simulink model "hil"  (R2025b)
settings: Solver=ode2  StartTime=0.0  StopTime=100  FixedStep=0.0025  RelTol=1e-3
undefined symbols (not defined in the file or in its folder): LF
libraries: instrumentseriallib x3
settings Model: SimulationMode=accelerator  PauseTimes=16  Creator=joedo  LastModifiedBy=trist
settings SFSimCC: SimHardwareAcceleration=native

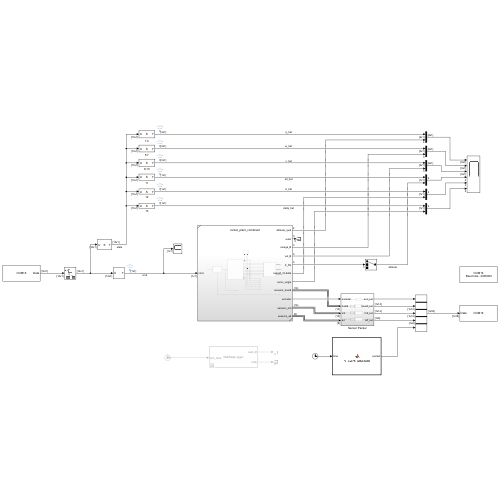
[thumbnail: Simulink's stored preview of the top-level diagram]
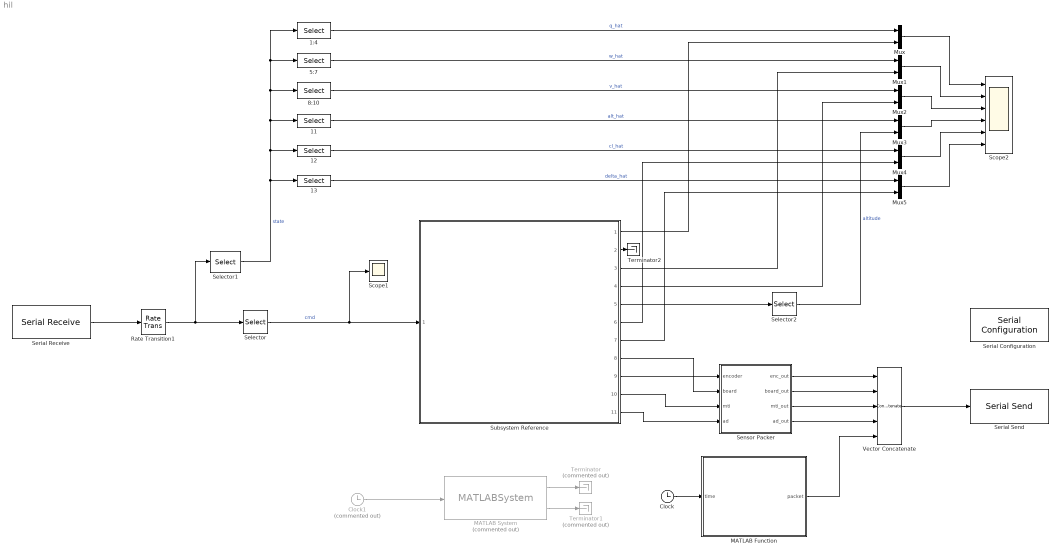
== system hil ==
  11 : Selector  InputPortWidth=13  IndexOptions=Index vector (dialog)  Indices=[11]  OutputSizes=1
  12 : Selector  InputPortWidth=13  IndexOptions=Index vector (dialog)  Indices=[12]  OutputSizes=1
  13 : Selector  InputPortWidth=13  IndexOptions=Index vector (dialog)  Indices=[13]  OutputSizes=1
  1:4 : Selector  InputPortWidth=13  IndexOptions=Index vector (dialog)  Indices=[1:4]  OutputSizes=1
  5:7 : Selector  InputPortWidth=13  IndexOptions=Index vector (dialog)  Indices=[5:7]  OutputSizes=1
  8:10 : Selector  InputPortWidth=13  IndexOptions=Index vector (dialog)  Indices=[8:10]  OutputSizes=1
  Clock : Clock
  Clock1 : Clock  Commented=on
  MATLAB Function : MATLAB Function  TreatAsAtomicUnit=on
  MATLAB System : MATLABSystem  Commented=on  System=WallStepLogger  Ts=0.0025  MaxSamples=50000  FileName=wall_step_log.mat  SimulateUsing=Code generation
      mask Type: WallStepLogger
  Mux{,1..5} (6 alike) : Mux  Inputs=2
  Rate Transition1 : RateTransition  OutPortSampleTime=0.01
  Scope1 : Scope
      settings: ActiveDisplayYMinimum=-1  ActiveDisplayYMaximum=1  DataLoggingVariableName=proccmd
  Scope2 : Scope  NumInputPorts=6
      settings: ActiveDisplayString=6  ActiveDisplayYMinimum=-0.00021816615649929114  ActiveDisplayYMaximum=0.0019634954084936209  DataLoggingVariableName=ScopeData9
  Selector : Selector  InputPortWidth=14  IndexOptions=Index vector (dialog)  Indices=[1]  OutputSizes=1
  Selector1 : Selector  InputPortWidth=14  IndexOptions=Index vector (dialog)  Indices=[2:14]  OutputSizes=1
  Selector2 : Selector  InputPortWidth=3  IndexOptions=Index vector (dialog)  Indices=[1]  OutputSizes=1
  Sensor Packer : Subsystem
  Serial Configuration : instrumentseriallib/Serial Configuration  Priority=-200000  PortSel=COM16  Port=COM16  ComPort=COM16  BaudRate=2000000  DataBits=8  Parity=none  StopBits=1  ByteOrder=little-endian  FlowControl=none  Timeout=10  SimulateUsing=Interpreted execution  BlockInModel=on  aMode=1
  Serial Receive : instrumentseriallib/Serial Receive  Priority=1  PortSel=COM16  Port=COM16  ComPort=COM16  DataType=double  SaveDataType=uint8  ToggleHeader=on  Header=[111, 114, 122, 33]  ToggleDataSize=on  DataSize=[14]  ToggleTerminator=on  Terminator=LF ('\n')  CustomTerminator=[]  InputFormat=Column major  EnableBlockingMode=on  ActionDataUnavailable=Output last received value  ActionWhenDataUnavailable=Output last received value  CustomValue=0  SampleTime=0.0025  SimulateUsing=Interpreted execution  BlockInModel=on  aMode=1  LibraryInUse=instrumentlib
  Serial Send : instrumentseriallib/Serial Send  Priority=1  PortSel=COM16  Port=COM16  ComPort=COM16  Header=[111, 114, 122, 33]  Terminator=LF ('\n')  CustomTerminator=[]  EnableBlockingMode=off  SimulateUsing=Interpreted execution  BlockInModel=on  aMode=1
  Subsystem Reference : Subsystem  ReferencedSubsystem=rocket_plant_combined
  Terminator : Terminator  Commented=on
  Terminator1 : Terminator  Commented=on
  Terminator2 : Terminator
  Vector Concatenate : Concatenate  NumInputs=5
  wires:
  Vector Concatenate/1 -> Serial Send/1
  Selector/1 -> Scope1/1, Subsystem Reference/1  "cmd"
  Selector1/1 -> 13/1, 12/1, 11/1, 8:10/1, 5:7/1, 1:4/1  "state"
  1:4/1 -> Mux/1  "q_hat"
  5:7/1 -> Mux1/1  "w_hat"
  8:10/1 -> Mux2/1  "v_hat"
  11/1 -> Mux3/1  "alt_hat"
  12/1 -> Mux4/1  "cl_hat"
  13/1 -> Mux5/1  "delta_hat"
  Subsystem Reference/1 -> Mux/2
  Subsystem Reference/3 -> Mux1/2
  Subsystem Reference/4 -> Mux2/2
  Subsystem Reference/5 -> Selector2/1
  Selector2/1 -> Mux3/2  "altitude"
  Subsystem Reference/6 -> Mux4/2
  Subsystem Reference/7 -> Mux5/2
  Mux/1 -> Scope2/1
  Mux1/1 -> Scope2/2
  Mux2/1 -> Scope2/3
  Mux3/1 -> Scope2/4
  Mux4/1 -> Scope2/5
  Mux5/1 -> Scope2/6
  Rate Transition1/1 -> Selector1/1, Selector/1
  Clock/1 -> MATLAB Function/1(time)
  MATLAB Function/1(packet) -> Vector Concatenate/5
  Serial Receive/1 -> Rate Transition1/1
  Clock1/1 -> MATLAB System/1
  MATLAB System/1 -> Terminator/1
  MATLAB System/2 -> Terminator1/1
  Subsystem Reference/2 -> Terminator2/1
  Sensor Packer/2(board_out) -> Vector Concatenate/2
  Sensor Packer/1(enc_out) -> Vector Concatenate/1
  Sensor Packer/3(mti_out) -> Vector Concatenate/3
  Sensor Packer/4(ad_out) -> Vector Concatenate/4
  Subsystem Reference/9 -> Sensor Packer/1(encoder)
  Subsystem Reference/8 -> Sensor Packer/2(board)
  Subsystem Reference/10 -> Sensor Packer/3(mti)
  Subsystem Reference/11 -> Sensor Packer/4(ad)

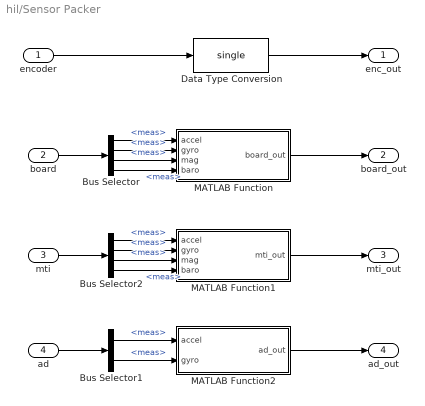
== system hil/Sensor Packer ==
  encoder : Inport
  board : Inport  Port=2
  mti : Inport  Port=3
  ad : Inport  Port=4
  Bus Selector : BusSelector  OutputSignals=board_accel.meas,board_gyro.meas,board_mag.meas,board_baro.meas
  Bus Selector1 : BusSelector  OutputSignals=ad_accel.meas,ad_gyro.meas
  Bus Selector2 : BusSelector  OutputSignals=mti_accel.meas,mti_gyro.meas,mti_mag.meas,mti_baro.meas
  Data Type Conversion : DataTypeConversion  OutDataTypeStr=single  SaturateOnIntegerOverflow=off  RndMeth=Floor
  MATLAB Function : MATLAB Function  TreatAsAtomicUnit=on
  MATLAB Function1 : MATLAB Function  TreatAsAtomicUnit=on
  MATLAB Function2 : MATLAB Function  TreatAsAtomicUnit=on
  enc_out : Outport
  board_out : Outport  Port=2
  mti_out : Outport  Port=3
  ad_out : Outport  Port=4
  wires:
  Data Type Conversion/1 -> enc_out/1
  encoder/1 -> Data Type Conversion/1
  board/1 -> Bus Selector/1
  Bus Selector/1 -> MATLAB Function/1(accel)  "<meas>"
  Bus Selector/2 -> MATLAB Function/2(gyro)  "<meas>"
  Bus Selector/3 -> MATLAB Function/3(mag)  "<meas>"
  Bus Selector/4 -> MATLAB Function/4(baro)  "<meas>"
  MATLAB Function/1(board_out) -> board_out/1
  MATLAB Function1/1(mti_out) -> mti_out/1
  Bus Selector2/1 -> MATLAB Function1/1(accel)  "<meas>"
  Bus Selector2/2 -> MATLAB Function1/2(gyro)  "<meas>"
  Bus Selector2/3 -> MATLAB Function1/3(mag)  "<meas>"
  Bus Selector2/4 -> MATLAB Function1/4(baro)  "<meas>"
  mti/1 -> Bus Selector2/1
  MATLAB Function2/1(ad_out) -> ad_out/1
  Bus Selector1/1 -> MATLAB Function2/1(accel)  "<meas>"
  Bus Selector1/2 -> MATLAB Function2/2(gyro)  "<meas>"
  ad/1 -> Bus Selector1/1

== matlab function hil/MATLAB Function ==
  settings: updateMethod=DISCRETE  sampleTime=0.0025
  data: time input; packet output
function packet  = hil_event_scheduler(time)

    t_hold = 0.1;
    
    % Command IDs
    CMD_NONE       = 0;
    CMD_LAUNCH     = 1;
    CMD_IGNITER    = 2;
    CMD_PAD_FILTER = 3;
    
    % Event schedule
    event_times = [10.0, 28.0, 30.0];   % seconds
    
    event_cmds = [ ...
        CMD_PAD_FILTER, ...
        CMD_IGNITER, ...
        CMD_LAUNCH ...
    ];
    
    cmd_id = CMD_NONE;
    
    % Send at most one event per timestep
    for k = 1:3
        if time > event_times(k) && time < (event_times(k) + t_hold)
            cmd_id = event_cmds(k);
        end
    end
    
    packet = single(cmd_id);

end

== matlab function hil/Sensor Packer/MATLAB Function ==
  data: accel input; board_out output; gyro input; mag input; baro input
function board_out = board_parse(accel, gyro, mag, baro)
    
    persistent k

    if isempty(k)
        k = 3;
    end

    if k <= 0
        stat_mag = 1;
        stat_baro = 1;
        k = 3;
    else
        stat_mag = 0;
        stat_baro = 0;
        k = k - 1;
    end


    board_out = zeros(1, 14, 'single');
    board_out(1:3) = accel;
    board_out(4) = 1; % accel status
    board_out(5:7) = gyro;
    board_out(8) = 1;
    board_out(9:11) = mag;
    board_out(12) = stat_mag;
    board_out(13) = baro;
    board_out(14) = stat_baro;

end

== matlab function hil/Sensor Packer/MATLAB Function1 ==
  data: accel input; mti_out output; gyro input; mag input; baro input
function mti_out = mti_parse(accel, gyro, mag, baro)
    
    persistent k

    if isempty(k)
        k = 3;
    end

    if k <= 0
        stat_mag = 1;
        stat_baro = 1;
        k = 3;
    else
        stat_mag = 0;
        stat_baro = 0;
        k = k - 1;
    end


    mti_out = zeros(1, 14, 'single');
    mti_out(1:3) = accel;
    mti_out(4) = 1; % accel status
    mti_out(5:7) = gyro;
    mti_out(8) = 1;
    mti_out(9:11) = mag;
    mti_out(12) = stat_mag;
    mti_out(13) = baro;
    mti_out(14) = stat_baro;

end

== matlab function hil/Sensor Packer/MATLAB Function2 ==
  data: accel input; ad_out output; gyro input
function ad_out = ad_parse(accel, gyro)

    ad_out = zeros(1, 8, 'single');
    ad_out(1:3) = accel;
    ad_out(4) = 1; % accel status
    ad_out(5:7) = gyro;
    ad_out(8) = 1;

end
